simulink model "chap8_14sim"  (Simulink 7.7)
settings: Solver=ode45  StartTime=0.0  StopTime=10  FixedStep=0.001  RelTol=1e-3
settings Model: Creator=hp  LastModifiedBy=ljk
settings DataIOCC: SignalLoggingName=sigsOut
settings OptimizationCC: InitFltsAndDblsToZero=on
settings DebuggingCC: SaveWithParameterizedLinksMsg=none  SignalResolutionControl=TryResolveAllWithWarning  SolverPrmCheckMsg=none  MultiTaskDSMMsg=warning  MultiTaskCondExecSysMsg=none  StrictBusMsg=Warning
settings HardwareCC: TargetUnknown=on
settings RTWCC: IncludeERTFirstTime=on
settings GRTTargetCC: TargetFcnLib=ansi_tfl_tmw.mat

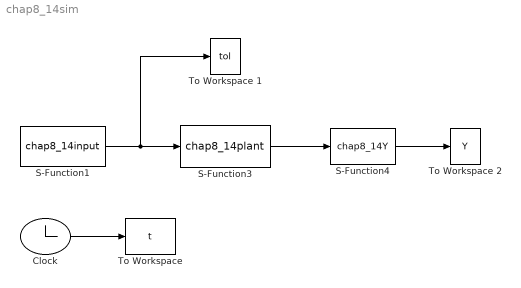
== system chap8_14sim ==
  Clock : Clock
      settings: Decimation=10
  S-Function1 : S-Function  FunctionName=chap8_14input  EnableBusSupport=off
  S-Function3 : S-Function  FunctionName=chap8_14plant  EnableBusSupport=off
  S-Function4 : S-Function  FunctionName=chap8_14Y  EnableBusSupport=off
  To Workspace : ToWorkspace  VariableName=t  SampleTime=-1  SaveFormat=Array
  To Workspace 1 : ToWorkspace  VariableName=tol  SampleTime=-1  SaveFormat=Array
  To Workspace 2 : ToWorkspace  VariableName=Y  SampleTime=-1  SaveFormat=Array
  wires:
  Clock/1 -> To Workspace/1
  S-Function1/1 -> S-Function3/1, To Workspace 1/1
  S-Function3/1 -> S-Function4/1
  S-Function4/1 -> To Workspace 2/1
